simulink subsystem "DYNAMICS"  (R2025b)
settings: Solver=VariableStepAuto  StartTime=0.0  StopTime=10.0  RelTol=1e-3
settings Model: Creator=antoniohernandez-rodiciomateos  LastModifiedBy=antoniohernandez-rodiciomateos

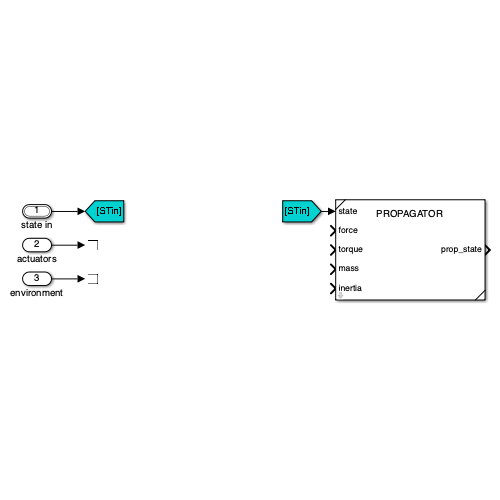
[thumbnail: Simulink's stored preview of the top-level diagram]
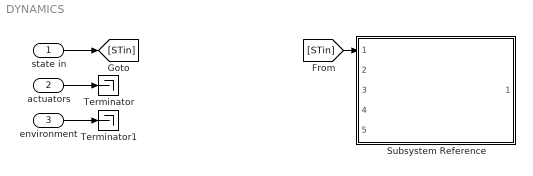
== system DYNAMICS ==
  state in : Inport  OutDataTypeStr=Bus: state_bus
  actuators : Inport  Port=2
  environment : Inport  Port=3
  Subsystem Reference : Subsystem  ReferencedSubsystem=PROPAGATOR  quatConv=q4 (scalar last)  forcesFrame=Inertial  r0=simData.ic.r0  v0=simData.ic.v0  att0=simData.ic.att0  omg0=simData.ic.omg0
  Terminator : Terminator
  Terminator1 : Terminator
  wires:
  actuators/1 -> Terminator/1
  environment/1 -> Terminator1/1
  state in/1 -> [STin]
  [STin] -> Subsystem Reference/1
